simulink model "mo2_2"  (R2024b)
settings: Solver=VariableStepAuto  StartTime=0.0  StopTime=10.0  RelTol=1e-3
undefined symbols (not defined in the file): Kc
settings Model: Creator=24839  LastModifiedBy=24839

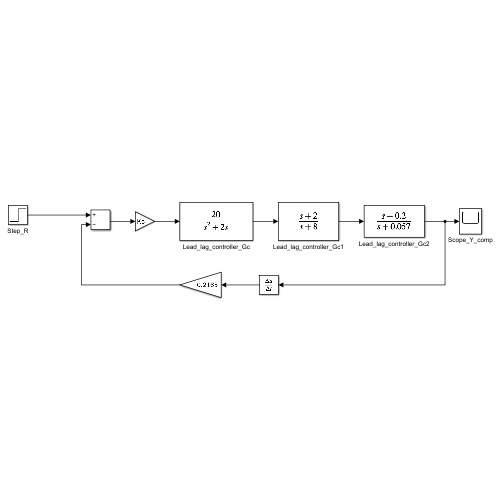
[thumbnail: Simulink's stored preview of the top-level diagram]
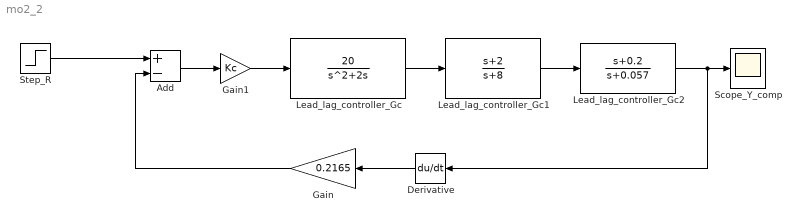
== system mo2_2 ==
  Add : Sum  Inputs=+-
  Derivative : Derivative
  Gain : Gain  Gain=0.2165
  Gain1 : Gain  Gain=Kc
  Lead_lag_controller_Gc : TransferFcn  Numerator=20  Denominator=[1 2 0]
  Lead_lag_controller_Gc1 : TransferFcn  Numerator=[1 2]  Denominator=[1 8]
  Lead_lag_controller_Gc2 : TransferFcn  Numerator=[1 0.2]  Denominator=[1 0.057]
  Scope_Y_comp : Scope
  Step_R : Step  Time=0  SampleTime=0
  wires:
  Step_R/1 -> Add/1
  Gain1/1 -> Lead_lag_controller_Gc/1
  Add/1 -> Gain1/1
  Lead_lag_controller_Gc/1 -> Lead_lag_controller_Gc1/1
  Lead_lag_controller_Gc1/1 -> Lead_lag_controller_Gc2/1
  Lead_lag_controller_Gc2/1 -> Derivative/1, Scope_Y_comp/1
  Derivative/1 -> Gain/1
  Gain/1 -> Add/2
